simulink model "HMC"  (R2026a)
settings: Solver=ode1  StopTime=inf  FixedStep=0.0001
PreLoadFcn:
  | %load('C:\Users\bme_master\Desktop\mot\mot_6_deneme.mat')
  | 
  | 
  | %load('C:\Users\bme_master\Desktop\mot\PRE_G''s.mat')
PostLoadFcn:
  | , if any(exist('dsrtsu_mdlpostloadfcn', 'file') ~= 0), dsrtsu_mdlpostloadfcn('Execute', bdroot); end,
InitFcn:
  | %motor_control_init_m
  | %clear all
  | %close all
  | %clc
  | b=1e-8
  | StepSize = 1e-4;
  | N=1e-17;
  | 
  | VLV_0 =0;%120; %120
  | VA_0 = 0;%300; %300
  | VRV_0 = 0;%130;
  | VP_0 = 0;%500;
  | VLA_0 = 0;%20;
  | VV_0=5000;
  | VRA_0=0;
  | 
  | 
  | QLV_0 = 0;
  | QLA_0 = 0;
  | QP_0 = 0;
  | 
  | bh = 0;
  | th =0;
  | 
  | X_0 = [VLV_0 VA_0 VV_0 VP_0  VLA_0  VRA_0 VRV_0];
  | 
  | 
  | V0 = 10;
  | 
  | K1=.0004;%0.0001
  | K2=0.0009;%0.0009
  | KA=1;%1
  | C1=0.000000003;%0.0000003
  | lambda=6000;%3000
  | X_00 = [VLV_0 VA_0 VV_0 VRV_0];
  | 
  | r2 = 0.05/2;
  | A2 = pi*r2^2;
  | h2 = 0.63;
  | V2 = A2*h2;
  | 
  | 
  | r3 = 0.05/2;
  | A3 = pi*r3^2;
  | h3 = 0.63;
  | V3 = A3*h3;
  | 
  | 
  | rho = 997;
  | gg = 9.81;
  | %
  | init_min=0;
  | init_max=0;
  | %
  | PWM_Period =  StepSize;
  | PWM_Period_g1 = PWM_Period;
  | PWM_Period_g2 =PWM_Period;
  | PWM_Period_g3 = PWM_Period;
  | PWM_Period_g4 = PWM_Period;
  | PWM_Period_g5 = PWM_Period;
  | ... (+158 lines)
undefined symbols (not defined in the file or in its folder): Continuous, DiscIntNeverNeededParam, Time
libraries: powerlib_meascontrol x19, simulink x15, rti1202lib_adc_class1 x11, cstblocks x10, rti1202lib_dio_class1 x8, dspstat3 x3, rti1202lib_dac_class1 x1, dspswit3 x1, ctrlSharedLib x1, slpidlib x1, dsparch4 x1
(part 3 of 5)

== system HMC/Reference CVSs/Pm/PID ==
  s : Inport
  LTI System : cstblocks/LTI System  sys=tfa  IC=[]
  PID Controller : simulink/Continuous/PID Controller  Controller=PID  Form=Parallel  TimeDomain=Continuous-time  SampleTime=-1  IntegratorMethod=Forward Euler  FilterMethod=Forward Euler  ControllerParametersSource=internal  P=0  I=0.336541519886425  D=0  UseFilter=on  N=100  TunerSelectOption=Transfer Function Based (PID Tuner App)  InitialConditionSource=internal  InitialConditionForIntegrator=0  InitialConditionForFilter=0  DifferentiatorICPrevScaledInput=0  ExternalReset=none  TrackingMode=off  Kt=1  LimitOutput=off  UpperSaturationLimit=inf  LowerSaturationLimit=-inf  LinearizeAsGain=on  AntiWindupMode=none  Kb=1  POutMin=[]  POutMax=[]  IOutMin=[]  IOutMax=[]  DOutMin=[]  DOutMax=[]  NOutMin=[]  NOutMax=[]  SumOutMin=[]  SumOutMax=[]  SaturationOutMin=[]  SaturationOutMax=[]  PParamMin=[]  PParamMax=[]  IParamMin=[]  IParamMax=[]  DParamMin=[]  DParamMax=[]  NParamMin=[]  NParamMax=[]  KbParamMin=[]  KbParamMax=[]  KtParamMin=[]  KtParamMax=[]  KbOutMin=[]  KbOutMax=[]  KtOutMin=[]  KtOutMax=[]  IntegratorOutMin=[]  IntegratorOutMax=[]  FilterOutMin=[]  FilterOutMax=[]  SumI1OutMin=[]  SumI1OutMax=[]  SumI2OutMin=[]  SumI2OutMax=[]  SumI3OutMin=[]  SumI3OutMax=[]  SumI4OutMin=[]  SumI4OutMax=[]  SumDOutMin=[]  SumDOutMax=[]  DifferentiatorOutMin=[]  DifferentiatorOutMax=[]  FilterDiffOutCoefMin=[]  FilterDiffOutCoefMax=[]  ReciprocalOutMin=[]  ReciprocalOutMax=[]  SumDenOutMin=[]  SumDenOutMax=[]  SumNumOutMin=[]  SumNumOutMax=[]  DivideOutMin=[]  DivideOutMax=[]  IntegratorContinuousStateAttributes=''  IntegratorStateMustResolveToSignalObject=off  IntegratorRTWStateStorageClass=Auto  FilterContinuousStateAttributes=''  FilterStateMustResolveToSignalObject=off  FilterRTWStateStorageClass=Auto  ParallelPVariant=InternalParameters  IdealPVariant=Disabled  IVariant=InternalParameters  DVariant=InternalParameters  IntegratorVariant=Continuous  SatVariant=Disabled  AWVariant=Passthrough  PCopyVariant=Disabled  TRVariant=Disabled  FdbkBlocksVariant=Forward  IdealPFdbkVariant=Disabled  SatFdbkVariant=Disabled  DerivativeFilterVariant=ContFilter  NVariant=InternalParameters  NCopyVariant=Disabled  FilterICVariant=InternalICsFilter  IntegratorICVariant=InternalICs  ExternalResetVariant=Disabled  TRSumVariant=Passthrough  SumFdbkVariant=Disabled  SumVariant=Sum_PID
  Sum1 : Sum  Inputs=|+-
  To Workspace : ToWorkspace  VariableName=input  SampleTime=-1
  To Workspace1 : ToWorkspace  VariableName=output  SampleTime=-1
  E : Outport  VectorParamsAs1DForOutWhenUnconnected=off
  wires:
  LTI System/1 -> To Workspace1/1, E/1, Sum1/2
  Sum1/1 -> PID Controller/1
  s/1 -> Sum1/1
  PID Controller/1 -> LTI System/1, To Workspace/1

== system HMC/Reference CVSs/Pressures Flows and Volumes/Exercise ==
  note: y = 0,0167x 2 + 0,6667x + 180
  note: y = -0,0069x2 + 1,2813x + 30,375R² = 1
  note: y = -0,1479x 2 + 38,021x - 923,75
  note: y = 0,1417x 2 - 24,583x + 2165
  note: y = -0,0033x 2 + 0,8667x - 16
  HR1 : Inport
  Enable : EnablePort
  Add{1..10,18..19} (12 alike) : Sum
  Constant1 : Constant  Value=180
  Constant2 : Constant  Value=-923.75
  Constant20 : Constant  Value=0.5621
  Constant3 : Constant  Value=30.375
  Constant4 : Constant  Value=-16
  Constant5 : Constant  Value=2165
  Gain : Gain  Gain=1/10000
  Gain1 : Gain  Gain=0.0167
  Gain10 : Gain  Gain=0.1417
  Gain11 : Gain  Gain=-24.583
  Gain12 : Gain  Gain=1/1000
  Gain13 : Gain  Gain=-0.0069
  Gain14 : Gain  Gain=1.2813
  Gain15 : Gain  Gain=1/10000
  Gain2 : Gain  Gain=0.000003
  Gain3 : Gain  Gain=-0.0008
  Gain4 : Gain  Gain=0.6667
  Gain5 : Gain  Gain=1/10000
  Gain6 : Gain  Gain=-0.0033
  Gain7 : Gain  Gain=0.8667
  Gain8 : Gain  Gain=-0.1479
  Gain9 : Gain  Gain=38.021
  Mux : Mux  Inputs=5
  Product{1..5,15} (6 alike) : Product
  Output : Outport
  wires:
  Add19/1 -> Mux/5  "eA"
  Product15/1 -> Gain2/1
  Constant20/1 -> Add19/2
  Add18/1 -> Add19/1
  Gain3/1 -> Add18/2
  Gain2/1 -> Add18/1
  Constant1/1 -> Add2/2
  HR1/1 -> Product2/1, Gain9/1, Product2/2, Product4/1, Product4/2, Gain14/1, Product5/1, Product5/2, Product15/1, Product15/2, Gain3/1, Gain4/1, Product1/2, Product1/1, Gain11/1, Gain7/1, Product3/2, Product3/1
  Add1/1 -> Add2/1
  Product1/1 -> Gain1/1
  Gain1/1 -> Add1/1
  Gain4/1 -> Add1/2
  Mux/1 -> Output/1
  Gain10/1 -> Add9/1
  Constant5/1 -> Add10/2
  Gain11/1 -> Add9/2
  Add9/1 -> Add10/1
  Add3/1 -> Add6/1
  Gain9/1 -> Add3/2
  Gain8/1 -> Add3/1
  Product4/1 -> Gain13/1
  Add8/1 -> Gain12/1
  Gain12/1 -> Mux/3
  Add10/1 -> Gain15/1
  Constant3/1 -> Add8/2
  Gain13/1 -> Add7/1
  Constant4/1 -> Add5/2
  Add4/1 -> Add5/1
  Gain6/1 -> Add4/1
  Constant2/1 -> Add6/2
  Add6/1 -> Gain/1
  Add5/1 -> Gain5/1
  Product2/1 -> Gain8/1
  Add7/1 -> Add8/1
  Gain5/1 -> Mux/1
  Product3/1 -> Gain6/1
  Gain14/1 -> Add7/2
  Gain7/1 -> Add4/2
  Product5/1 -> Gain10/1
  Gain/1 -> Mux/2
  Gain15/1 -> Mux/4

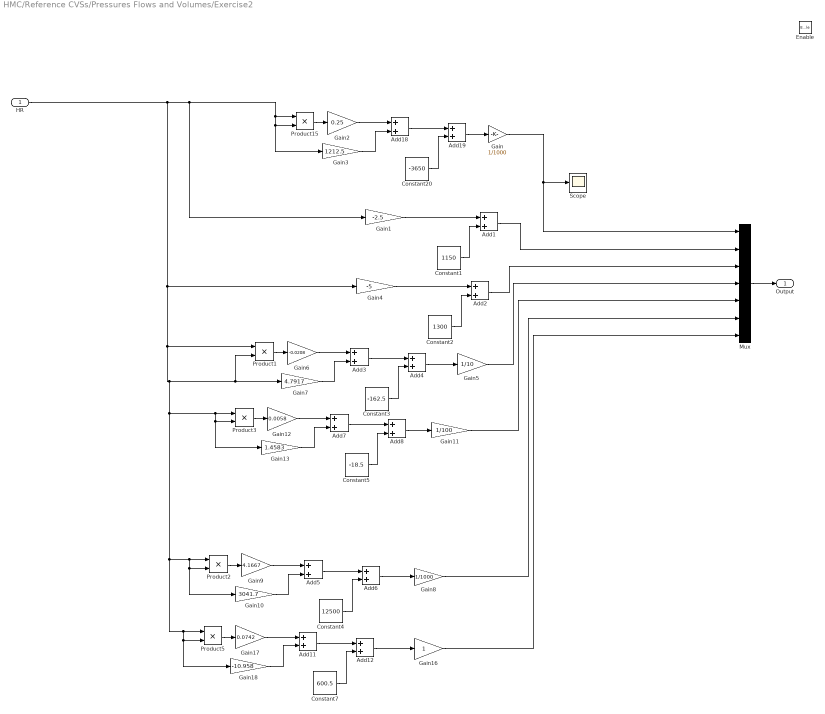
== system HMC/Reference CVSs/Pressures Flows and Volumes/Exercise2 ==
  HR : Inport
  Enable : EnablePort
  Add{1..8,11..12,18..19} (12 alike) : Sum
  Constant1 : Constant  Value=1150
  Constant2 : Constant  Value=1300
  Constant20 : Constant  Value=-3650
  Constant3 : Constant  Value=-162.5
  Constant4 : Constant  Value=12500
  Constant5 : Constant  Value=-18.5
  Constant7 : Constant  Value=600.5
  Gain : Gain  Gain=1/1000
  Gain1 : Gain  Gain=-2.5
  Gain10 : Gain  Gain=3041.7
  Gain11 : Gain  Gain=1/100
  Gain12 : Gain  Gain=0.0058
  Gain13 : Gain  Gain=1.4583
  Gain16 : Gain
  Gain17 : Gain  Gain=0.0742
  Gain18 : Gain  Gain=-10.958
  Gain2 : Gain  Gain=0.25
  Gain3 : Gain  Gain=1212.5
  Gain4 : Gain  Gain=-5
  Gain5 : Gain  Gain=1/10
  Gain6 : Gain  Gain=-0.0208
  Gain7 : Gain  Gain=4.7917
  Gain8 : Gain  Gain=1/1000
  Gain9 : Gain  Gain=4.1667
  Mux : Mux  Inputs=7
  Product{1..3,5,15} (5 alike) : Product
  Scope : Scope
      settings: ActiveDisplayYMinimum=60  ActiveDisplayYMaximum=80  DataLoggingVariableName=ScopeData9
  Output : Outport
  wires:
  Gain9/1 -> Add5/1
  Product2/1 -> Gain9/1
  Add5/1 -> Add6/1
  Gain8/1 -> Mux/6
  Gain10/1 -> Add5/2
  Constant4/1 -> Add6/2
  Add6/1 -> Gain8/1
  Add3/1 -> Add4/1
  Add4/1 -> Gain5/1
  Gain6/1 -> Add3/1
  Product1/1 -> Gain6/1
  Gain5/1 -> Mux/4
  Gain7/1 -> Add3/2
  Constant3/1 -> Add4/2
  Constant2/1 -> Add2/2
  Add2/1 -> Mux/3
  Gain4/1 -> Add2/1
  Gain1/1 -> Add1/1
  Constant1/1 -> Add1/2
  Add1/1 -> Mux/2
  Add18/1 -> Add19/1
  Add19/1 -> Gain/1
  Gain3/1 -> Add18/2
  Product15/1 -> Gain2/1
  Constant20/1 -> Add19/2
  Gain/1 -> Scope/1, Mux/1
  Gain2/1 -> Add18/1
  Mux/1 -> Output/1
  Gain12/1 -> Add7/1
  Add7/1 -> Add8/1
  Constant5/1 -> Add8/2
  Product3/1 -> Gain12/1
  Add8/1 -> Gain11/1
  Gain11/1 -> Mux/5
  Gain13/1 -> Add7/2
  Product5/1 -> Gain17/1
  Add11/1 -> Add12/1
  Constant7/1 -> Add12/2
  Add12/1 -> Gain16/1
  HR/1 -> Gain3/1, Product15/2, Product15/1, Gain1/1, Gain7/1, Product1/2, Gain10/1, Product2/2, Product2/1, Product5/1, Product5/2, Gain18/1, Gain13/1, Product3/2, Product3/1, Product1/1, Gain4/1
  Gain17/1 -> Add11/1
  Gain16/1 -> Mux/7
  Gain18/1 -> Add11/2

== system HMC/Reference CVSs/Pressures Flows and Volumes/HF ==
  note: y = 0,5x + 40
  note: y = - 0,3333x + 130
  note: y = 0,0128x 2 - 1,9167x + 179
  note: y = -0,0189x 2 + 3,5x + 78
  note: y = 0,4333x + 14
  note: eV
  note: eRA
  note: eLA
  note: eP
  note: eA
  HR : Inport
  Enable : EnablePort
  Add{1..4,6,8,19} (7 alike) : Sum
  Constant1 : Constant  Value=78
  Constant2 : Constant  Value=179
  Constant20 : Constant  Value=14
  Constant3 : Constant  Value=130
  Constant4 : Constant  Value=40
  Gain : Gain  Gain=1/1000
  Gain1 : Gain  Gain=1/10000
  Gain11 : Gain  Gain=-0.3333
  Gain13 : Gain  Gain=0.5
  Gain3 : Gain  Gain=0.4333
  Gain4 : Gain  Gain=-0.0189
  Gain5 : Gain  Gain=3.5
  Gain6 : Gain  Gain=1/1000
  Gain7 : Gain  Gain=0.0128
  Gain8 : Gain  Gain=-1.9167
  Gain9 : Gain  Gain=1/1000
  Multiply : Gain  Gain=1/100
  Mux : Mux  Inputs=5
  Product1 : Product
  Product2 : Product
  Output : Outport
  wires:
  Gain3/1 -> Add19/1
  Constant20/1 -> Add19/2
  Gain1/1 -> Mux/1
  Add19/1 -> Gain1/1
  Add1/1 -> Add2/1
  Gain/1 -> Mux/2
  Product1/1 -> Gain4/1
  Gain4/1 -> Add1/1
  Add2/1 -> Gain/1
  Gain5/1 -> Add1/2
  Constant1/1 -> Add2/2
  Add3/1 -> Add4/1
  Gain7/1 -> Add3/1
  Gain8/1 -> Add3/2
  Add4/1 -> Gain6/1
  Constant2/1 -> Add4/2
  Product2/1 -> Gain7/1
  Gain6/1 -> Mux/3
  Add6/1 -> Gain9/1
  Gain11/1 -> Add6/1
  Constant3/1 -> Add6/2
  Gain9/1 -> Mux/4
  Mux/1 -> Output/1
  Multiply/1 -> Mux/5
  Add8/1 -> Multiply/1
  Constant4/1 -> Add8/2
  Gain13/1 -> Add8/1
  HR/1 -> Product1/1, Product1/2, Gain5/1, Gain13/1, Gain11/1, Product2/1, Product2/2, Gain8/1, Gain3/1

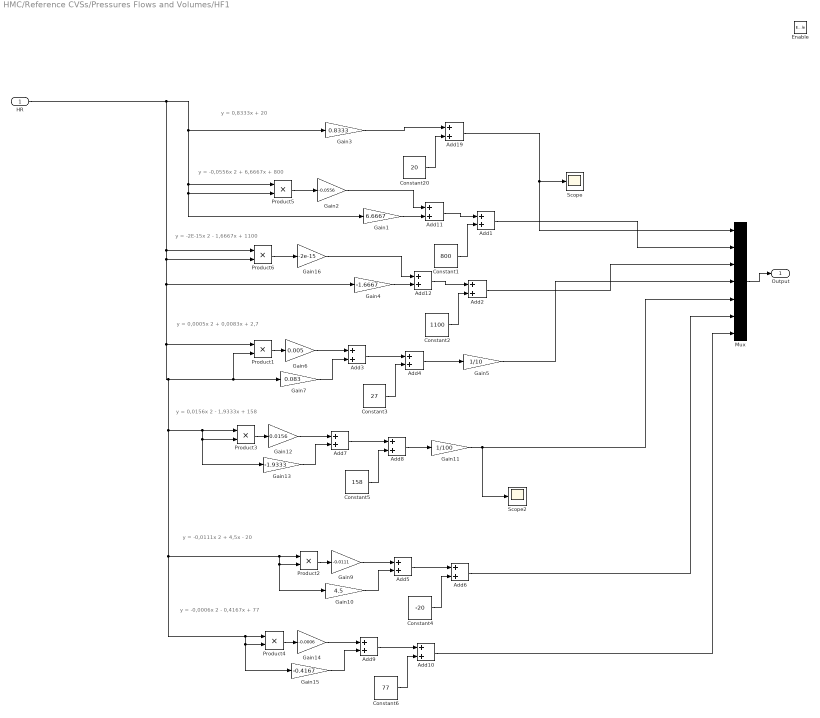
== system HMC/Reference CVSs/Pressures Flows and Volumes/HF1 ==
  note: y = -0,0111x 2 + 4,5x - 20
  note: y = -2E-15x 2 - 1,6667x + 1100
  note: y = 0,8333x + 20
  note: y = 0,0005x 2 + 0,0083x + 2,7
  note: y = -0,0556x 2 + 6,6667x + 800
  note: y = 0,0156x 2 - 1,9333x + 158
  note: y = -0,0006x 2 - 0,4167x + 77
  HR : Inport
  Enable : EnablePort
  Add{1..12,19} (13 alike) : Sum
  Constant1 : Constant  Value=800
  Constant2 : Constant  Value=1100
  Constant20 : Constant  Value=20
  Constant3 : Constant  Value=27
  Constant4 : Constant  Value=-20
  Constant5 : Constant  Value=158
  Constant6 : Constant  Value=77
  Gain1 : Gain  Gain=6.6667
  Gain10 : Gain  Gain=4.5
  Gain11 : Gain  Gain=1/100
  Gain12 : Gain  Gain=0.0156
  Gain13 : Gain  Gain=-1.9333
  Gain14 : Gain  Gain=-0.0006
  Gain15 : Gain  Gain=-0.4167
  Gain16 : Gain  Gain=-2e-15
  Gain2 : Gain  Gain=-0.0556
  Gain3 : Gain  Gain=0.8333
  Gain4 : Gain  Gain=-1.6667
  Gain5 : Gain  Gain=1/10
  Gain6 : Gain  Gain=0.005
  Gain7 : Gain  Gain=0.083
  Gain9 : Gain  Gain=-0.0111
  Mux : Mux  Inputs=7
  Product{1..6} (6 alike) : Product
  Scope : Scope
      settings: ActiveDisplayYMinimum=60  ActiveDisplayYMaximum=80  DataLoggingVariableName=ScopeData4
  Scope2 : Scope
      settings: ActiveDisplayYMinimum=0.88246  ActiveDisplayYMaximum=1.08246  DataLoggingVariableName=ScopeData5
  Output : Outport
  wires:
  Add6/1 -> Mux/6
  Product6/1 -> Gain16/1
  Product5/1 -> Gain2/1
  Gain1/1 -> Add11/2
  Add4/1 -> Gain5/1
  Product4/1 -> Gain14/1
  Gain13/1 -> Add7/2
  Constant6/1 -> Add10/2
  Gain12/1 -> Add7/1
  Gain16/1 -> Add12/1
  Add2/1 -> Mux/3
  Constant3/1 -> Add4/2
  Gain10/1 -> Add5/2
  Gain9/1 -> Add5/1
  Gain11/1 -> Mux/5, Scope2/1
  Product1/1 -> Gain6/1
  Add8/1 -> Gain11/1
  Gain7/1 -> Add3/2
  Add7/1 -> Add8/1
  Product2/1 -> Gain9/1
  Constant4/1 -> Add6/2
  Gain6/1 -> Add3/1
  Constant2/1 -> Add2/2
  Mux/1 -> Output/1
  Constant1/1 -> Add1/2
  Product3/1 -> Gain12/1
  Gain14/1 -> Add9/1
  Add9/1 -> Add10/1
  Gain15/1 -> Add9/2
  Gain3/1 -> Add19/1
  Add19/1 -> Mux/1, Scope/1
  Constant5/1 -> Add8/2
  Gain5/1 -> Mux/4
  Add10/1 -> Mux/7
  Add11/1 -> Add1/1
  Add3/1 -> Add4/1
  Add1/1 -> Mux/2
  Gain4/1 -> Add12/2
  Constant20/1 -> Add19/2
  Gain2/1 -> Add11/1
  Add5/1 -> Add6/1
  Add12/1 -> Add2/1
  HR/1 -> Product6/1, Product6/2, Gain4/1, Product1/1, Gain13/1, Product3/2, Product3/1, Gain15/1, Product4/2, Product4/1, Product2/1, Product2/2, Gain10/1, Product1/2, Gain7/1, Product5/1, Gain1/1, Product5/2, Gain3/1

== system HMC/Reference CVSs/Pressures Flows and Volumes/Rest ==
  note: eC
  note: y = -0,0033x 2 + 0,8667x - 16
  note: eRA
  note: eLA
  note: eP
  note: y = 0,1417x 2 - 24,583x + 2165
  note: y = -0,0069x2 + 1,2813x + 30,375R² = 1
  note: y = -0,1479x 2 + 38,021x - 923,75
  note: y = 0,5x + 40
  note: eV
  HR : Inport
  Input : Inport  Port=2
  Enable : EnablePort
  Add{1..7,18..19} (9 alike) : Sum
  Constant1 : Constant  Value=-923.75
  Constant2 : Constant  Value=30.375
  Constant20 : Constant  Value=-16
  Constant3 : Constant  Value=2165
  Constant4 : Constant  Value=40
  Gain : Gain  Gain=1/10000
  Gain1 : Gain  Gain=1/10000
  Gain10 : Gain  Gain=0.1417
  Gain11 : Gain  Gain=-24.583
  Gain12 : Gain  Gain=1/100
  Gain13 : Gain  Gain=0.5
  Gain2 : Gain  Gain=-0.0033
  Gain3 : Gain  Gain=0.8667
  Gain4 : Gain  Gain=-0.1479
  Gain5 : Gain  Gain=38.021
  Gain6 : Gain  Gain=1/1000
  Gain7 : Gain  Gain=-0.0069
  Gain8 : Gain  Gain=1.2813
  Gain9 : Gain  Gain=1/10000
  Mux : Mux  Inputs=5
  Product{1..3,15} (4 alike) : Product
  Output : Outport
  wires:
  Gain3/1 -> Add18/2
  Product15/1 -> Gain2/1
  Add19/1 -> Gain1/1
  Constant20/1 -> Add19/2
  Gain2/1 -> Add18/1
  Add18/1 -> Add19/1
  Gain1/1 -> Mux/1
  Gain6/1 -> Mux/3
  Mux/1 -> Output/1
  Gain/1 -> Mux/2
  Gain9/1 -> Mux/4
  Gain4/1 -> Add1/1
  Gain5/1 -> Add1/2
  Constant1/1 -> Add2/2
  Add2/1 -> Gain/1
  Add1/1 -> Add2/1
  Product1/1 -> Gain4/1
  Gain7/1 -> Add3/1
  Constant2/1 -> Add4/2
  Add3/1 -> Add4/1
  Add4/1 -> Gain6/1
  Gain8/1 -> Add3/2
  Product2/1 -> Gain7/1
  HR/1 -> Product1/1, Gain5/1, Product1/2, Product2/1, Product2/2, Gain8/1, Product3/1, Product3/2, Gain11/1, Gain3/1, Product15/2, Product15/1
  Add5/1 -> Add6/1
  Product3/1 -> Gain10/1
  Constant3/1 -> Add6/2
  Gain10/1 -> Add5/1
  Gain11/1 -> Add5/2
  Add6/1 -> Gain9/1
  Add7/1 -> Gain12/1
  Constant4/1 -> Add7/2
  Gain13/1 -> Add7/1
  Gain12/1 -> Mux/5  "eA"
  Input/1 -> Gain13/1

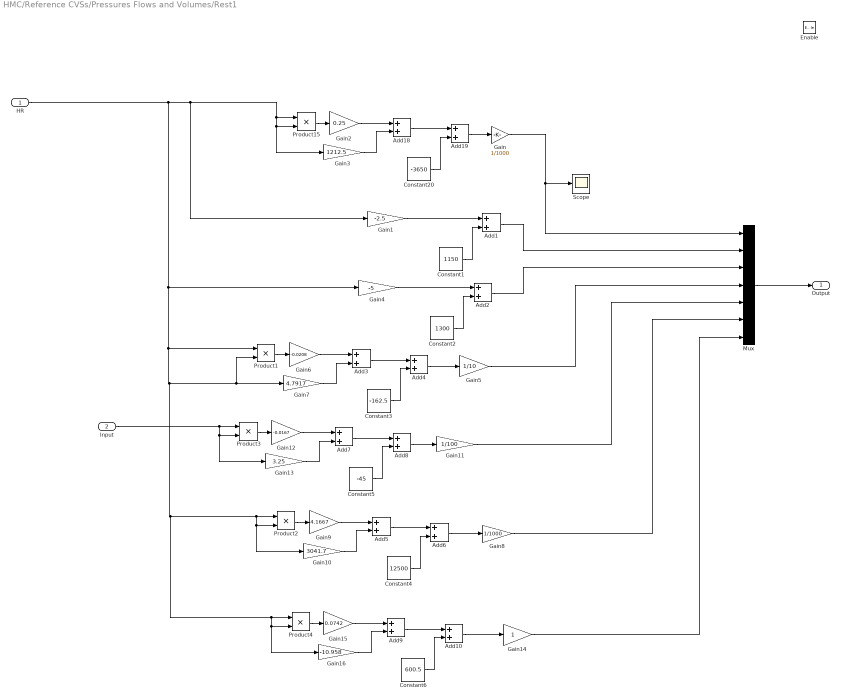
== system HMC/Reference CVSs/Pressures Flows and Volumes/Rest1 ==
  HR : Inport
  Input : Inport  Port=2
  Enable : EnablePort
  Add{1..10,18..19} (12 alike) : Sum
  Constant1 : Constant  Value=1150
  Constant2 : Constant  Value=1300
  Constant20 : Constant  Value=-3650
  Constant3 : Constant  Value=-162.5
  Constant4 : Constant  Value=12500
  Constant5 : Constant  Value=-45
  Constant6 : Constant  Value=600.5
  Gain : Gain  Gain=1/1000
  Gain1 : Gain  Gain=-2.5
  Gain10 : Gain  Gain=3041.7
  Gain11 : Gain  Gain=1/100
  Gain12 : Gain  Gain=-0.0167
  Gain13 : Gain  Gain=3.25
  Gain14 : Gain
  Gain15 : Gain  Gain=0.0742
  Gain16 : Gain  Gain=-10.958
  Gain2 : Gain  Gain=0.25
  Gain3 : Gain  Gain=1212.5
  Gain4 : Gain  Gain=-5
  Gain5 : Gain  Gain=1/10
  Gain6 : Gain  Gain=-0.0208
  Gain7 : Gain  Gain=4.7917
  Gain8 : Gain  Gain=1/1000
  Gain9 : Gain  Gain=4.1667
  Mux : Mux  Inputs=7
  Product{1..4,15} (5 alike) : Product
  Scope : Scope
      settings: ActiveDisplayYMinimum=60  ActiveDisplayYMaximum=80  DataLoggingVariableName=ScopeData9
  Output : Outport
  wires:
  Mux/1 -> Output/1
  Gain2/1 -> Add18/1
  Gain/1 -> Mux/1, Scope/1
  Constant20/1 -> Add19/2
  Product15/1 -> Gain2/1
  Gain3/1 -> Add18/2
  Add19/1 -> Gain/1
  Add18/1 -> Add19/1
  Add1/1 -> Mux/2
  Constant1/1 -> Add1/2
  Gain1/1 -> Add1/1
  Gain4/1 -> Add2/1
  Add2/1 -> Mux/3
  Constant2/1 -> Add2/2
  Constant3/1 -> Add4/2
  Gain7/1 -> Add3/2
  Gain5/1 -> Mux/4
  Product1/1 -> Gain6/1
  Gain6/1 -> Add3/1
  Add4/1 -> Gain5/1
  Add3/1 -> Add4/1
  Add6/1 -> Gain8/1
  Constant4/1 -> Add6/2
  Gain10/1 -> Add5/2
  Gain8/1 -> Mux/6
  Add5/1 -> Add6/1
  Product2/1 -> Gain9/1
  Gain9/1 -> Add5/1
  Gain13/1 -> Add7/2
  Add7/1 -> Add8/1
  Product3/1 -> Gain12/1
  Constant5/1 -> Add8/2
  Add8/1 -> Gain11/1
  Gain12/1 -> Add7/1
  Input/1 -> Product3/1, Product3/2, Gain13/1
  Gain11/1 -> Mux/5
  Product4/1 -> Gain15/1
  Add9/1 -> Add10/1
  Constant6/1 -> Add10/2
  Add10/1 -> Gain14/1
  HR/1 -> Gain4/1, Product1/1, Product4/1, Product4/2, Gain16/1, Product2/1, Product2/2, Gain10/1, Product1/2, Gain7/1, Gain1/1, Product15/1, Product15/2, Gain3/1
  Gain15/1 -> Add9/1
  Gain14/1 -> Mux/7
  Gain16/1 -> Add9/2

== system HMC/Reference CVSs/Pressures Flows and Volumes/Subsystem13 ==
  note: y = 0,0083x 2 - 0,9167x + 40
  note: y = 0,1944x 2 - 28,333x + 1100
  Add{1..2,18..19} (4 alike) : Sum
  Constant1 : Constant  Value=40
  Constant20 : Constant  Value=1100
  Display : Display
  Gain : Gain  Gain=1/10
  Gain2 : Gain  Gain=0.1944
  Gain3 : Gain  Gain=-28.333
  Gain4 : Gain  Gain=0.0083
  Gain5 : Gain  Gain=-0.9167
  Product1 : Product
  Product15 : Product
  Scope : Scope
      settings: ActiveDisplayYMinimum=8.99968  ActiveDisplayYMaximum=10.99968  DataLoggingVariableName=ScopeData2
  Scope1 : Scope
      settings: ActiveDisplayYMinimum=8.99968  ActiveDisplayYMaximum=10.99968
  Switch : Switch  Criteria=u2 > Threshold  SaturateOnIntegerOverflow=off  InputSameDT=off
  V0 : Outport
  wires:
  Add19/1 -> Gain/1
  Add18/1 -> Add19/1
  Gain3/1 -> Add18/2
  Product15/1 -> Gain2/1
  Constant20/1 -> Add19/2
  Gain2/1 -> Add18/1
  [HR] -> Product15/1, Product15/2, Gain3/1
  Gain/1 -> Switch/3, Scope/1
  Add2/1 -> Switch/1, Scope1/1
  [HR] -> Gain5/1, Product1/2, Product1/1
  Gain4/1 -> Add1/1
  Constant1/1 -> Add2/2
  Product1/1 -> Gain4/1
  Gain5/1 -> Add1/2
  Add1/1 -> Add2/1
  [Heart_Failure_On_Off] -> Switch/2
  Switch/1 -> Display/1, V0/1

== system HMC/Reference CVSs/Pressures Flows and Volumes/Subsystem5 ==
  In1 : Inport
  elv : Inport  Port=2
  erv : Inport  Port=3
  In4 : Inport  Port=4
  Switch : Switch  Criteria=u2 > Threshold  SaturateOnIntegerOverflow=off  InputSameDT=off
  Switch4 : Switch  Criteria=u2 > Threshold  SaturateOnIntegerOverflow=off  InputSameDT=off
  VolumesForVAD : Subsystem
  Out1 : Outport
  Output1 : Outport  Port=2
  wires:
  [QVAD] -> Switch4/2, Switch/2
  elv/1 -> VolumesForVAD/1(elv1)
  VolumesForVAD/2(Output1) -> Switch4/1
  erv/1 -> VolumesForVAD/2(erv1)
  VolumesForVAD/1(Output2) -> Switch/1
  In1/1 -> Switch/3
  Switch4/1 -> Output1/1
  Switch/1 -> Out1/1
  In4/1 -> Switch4/3

== system HMC/Reference CVSs/eLV/LV_e_min ==
  VLV : Inport
  Add : Sum  Inputs=+-
  Add1 : Sum  Inputs=+-
  Add2 : Sum
  Constant9 : Constant
  Display : Display
  Display1 : Display
  Exp : Math  SignedPower=on
  Product : Product
  Product1 : Product
  Real_CLV : Subsystem
  Subsystem1 : Subsystem
  Subsystem2 : Subsystem
  Subsystem5 : Subsystem
  Switch : Switch  Criteria=u2 > Threshold  SaturateOnIntegerOverflow=off  InputSameDT=off
  Switch1 : Switch  Criteria=u2 > Threshold  SaturateOnIntegerOverflow=off  InputSameDT=off
  Switch2 : Switch  Criteria=u2 > Threshold  SaturateOnIntegerOverflow=off  InputSameDT=off
  a_LV_Cons : Constant  Value=0.4641
  d_LV_Cons : Constant  Value=0.1235
  resting : Subsystem
  eLV_min_O : Outport
  tag scope: bLV=global, cLV=global
  wires:
  Add/1 -> Product1/2
  Product1/1 -> Exp/1
  Exp/1 -> Add1/1
  d_LV_Cons/1 -> Add2/2
  Product/1 -> Add2/1
  Add1/1 -> Product/2
  Constant9/1 -> Add1/2
  VLV/1 -> Add/1
  Add2/1 -> eLV_min_O/1
  a_LV_Cons/1 -> Product/1
  [Heart_Failure_On_Off] -> Switch/2
  Subsystem1/1(C_LV) -> Switch1/3
  [Heart_Failure_On_Off] -> Switch1/2
  Real_CLV/1(C_LV) -> Switch1/1
  Subsystem5/1(B_LV_HF) -> Switch/1
  [Exercise_On_Off] -> Switch2/2
  resting/1(B_LV) -> Switch2/3
  Subsystem2/1(B_LV) -> Switch2/1
  Switch/1 -> [bLV], Product1/1, Display/1
  Switch2/1 -> Switch/3
  Switch1/1 -> [cLV], Add/2, Display1/1

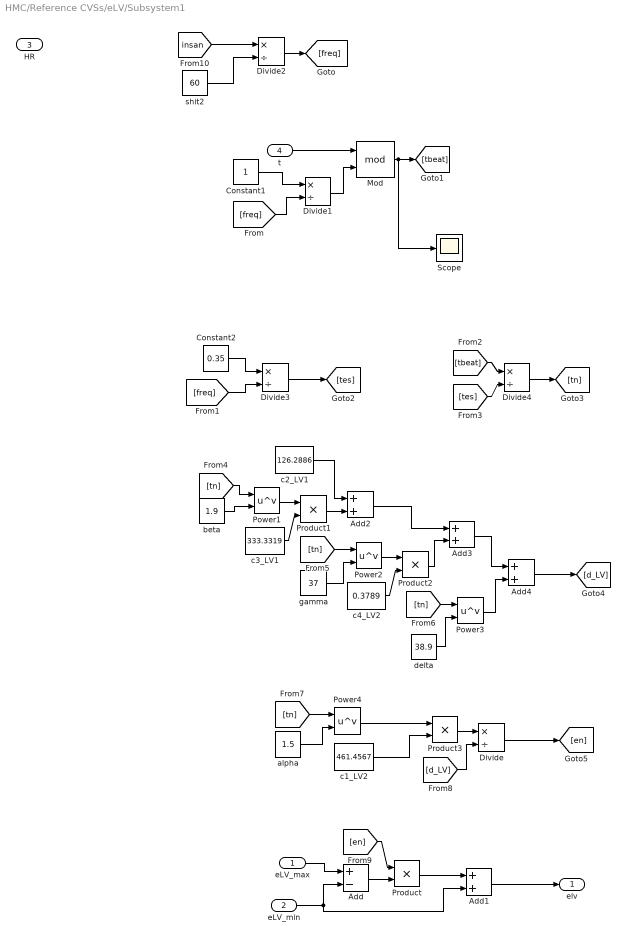
== system HMC/Reference CVSs/eLV/Subsystem1 ==
  eLV_max : Inport
  eLV_min : Inport  Port=2
  HR : Inport  Port=3
  t : Inport  Port=4
  Add : Sum  Inputs=+-
  Add{1..4} (4 alike) : Sum
  Constant1 : Constant
  Constant2 : Constant  Value=0.35
  Divide{,1..4} (5 alike) : Product  Inputs=*/  RndMeth=Zero  SaturateOnIntegerOverflow=on
  Mod : Math  Operator=mod  SignedPower=on
  Power{1..4} (4 alike) : Math  Operator=pow  SignedPower=on
  Product{,1..3} (4 alike) : Product
  Scope : Scope
      settings: ActiveDisplayYMinimum=-0.05357  ActiveDisplayYMaximum=0.43719  DataLoggingVariableName=ScopeData4
  alpha : Constant  Value=1.5
  beta : Constant  Value=1.9
  c1_LV2 : Constant  Value=461.4567
  c2_LV1 : Constant  Value=126.2886
  c3_LV1 : Constant  Value=333.3319
  c4_LV2 : Constant  Value=0.3789
  delta : Constant  Value=38.9
  gamma : Constant  Value=37
  "shit2 " : Constant  Value=60
  elv : Outport
  wires:
  Product/1 -> Add1/1
  Add/1 -> Product/2
  Add1/1 -> elv/1
  eLV_min/1 -> Add/2, Add1/2
  eLV_max/1 -> Add/1
  "shit2 "/1 -> Divide2/2
  Divide2/1 -> [freq]
  [freq] -> Divide1/2
  Constant1/1 -> Divide1/1
  Constant2/1 -> Divide3/1
  [freq] -> Divide3/2
  Divide3/1 -> [tes]
  [tbeat] -> Divide4/1
  [tes] -> Divide4/2
  Divide4/1 -> [tn]
  c2_LV1/1 -> Add2/1
  [tn] -> Power1/1
  beta/1 -> Power1/2
  Power1/1 -> Product1/1
  c3_LV1/1 -> Product1/2
  Product1/1 -> Add2/2
  Add2/1 -> Add3/1
  [tn] -> Power2/1
  gamma/1 -> Power2/2
  Power2/1 -> Product2/1
  c4_LV2/1 -> Product2/2
  Product2/1 -> Add3/2
  [tn] -> Power3/1
  delta/1 -> Power3/2
  Add3/1 -> Add4/1
  Power3/1 -> Add4/2
  Add4/1 -> [d_LV]
  [tn] -> Power4/1
  alpha/1 -> Power4/2
  Power4/1 -> Product3/1
  c1_LV2/1 -> Product3/2
  Product3/1 -> Divide/1
  Divide/1 -> [en]
  [d_LV] -> Divide/2
  [en] -> Product/1
  t/1 -> Mod/1
  Divide1/1 -> Mod/2
  Mod/1 -> Scope/1, [tbeat]
  [insan] -> Divide2/1

== system HMC/Reference CVSs/eLV/eLV1 ==
  note: y = 0,0027x 2 - 0,0767x + 24,76
  Add18 : Sum
  Add19 : Sum
  Constant20 : Constant  Value=24.76
  Gain1 : Gain  Gain=1/10
  Gain2 : Gain  Gain=0.0027
  Gain3 : Gain  Gain=-0.0767
  PID : Subsystem  Commented=on
  Product15 : Product
  Scope : Scope
      settings: ActiveDisplayYMinimum=2.20237  ActiveDisplayYMaximum=2.60692
  Stair Generator : powerlib_meascontrol/Pulse & Signal Generators/Stair Generator  Commented=on  t=[0,50,100,150]  e=[3.25,3.5,3.75,4]  Ts=stepsize
      settings: SourceProductName=Simscape Electrical
  Stair Generator1 : powerlib_meascontrol/Pulse & Signal Generators/Stair Generator  Commented=on  t=[100,200,300,400]  e=[3.25,3.5,3.75,4]  Ts=stepsize
      settings: SourceProductName=Simscape Electrical
  Output : Outport
  wires:
  Stair Generator1/1 -> PID/1(s)
  Add19/1 -> Gain1/1
  Gain2/1 -> Add18/1
  Gain3/1 -> Add18/2
  [HR] -> Product15/1, Product15/2, Gain3/1
  Add18/1 -> Add19/1
  Product15/1 -> Gain2/1
  Constant20/1 -> Add19/2
  Gain1/1 -> Scope/1, Output/1

== system HMC/Reference CVSs/eLV/eLVsick ==
  note: y = -0,0028x 2 + 0,9167x + 45
  Add18 : Sum
  Add19 : Sum
  Constant20 : Constant  Value=45
  Gain1 : Gain  Gain=1/100
  Gain2 : Gain  Gain=-0.0028
  Gain3 : Gain  Gain=0.9167
  Product15 : Product
  Scope : Scope
      settings: ActiveDisplayYMinimum=2.20237  ActiveDisplayYMaximum=2.60692  DataLoggingVariableName=ScopeData6
  Output : Outport
  wires:
  Product15/1 -> Gain2/1
  Gain1/1 -> Scope/1, Output/1
  Gain3/1 -> Add18/2
  Constant20/1 -> Add19/2
  Gain2/1 -> Add18/1
  [HR] -> Product15/1, Product15/2, Gain3/1
  Add18/1 -> Add19/1
  Add19/1 -> Gain1/1

== system HMC/Reference CVSs/eRV/RV_e_min ==
  VRV : Inport
  Add3 : Sum  Inputs=+-
  Add4 : Sum
  Constant13 : Constant
  Display1 : Display
  Exp1 : Math  SignedPower=on
  Product2 : Product
  Product3 : Product
  Switch1 : Switch  Criteria=u2 > Threshold  Threshold=0.9  SaturateOnIntegerOverflow=off  InputSameDT=off
  a_RV_Cons : Constant  Value=0.03752
  b_RV_Cons : Constant  Value=0.03776
  c_RV : Subsystem
  real_c_RV : Subsystem
  eRV_min_O : Outport
  tag scope: cRV=global
  wires:
  Constant13/1 -> Add4/2
  Product2/1 -> Exp1/1
  Add3/1 -> Product2/1
  VRV/1 -> Add3/1
  Exp1/1 -> Add4/1
  Add4/1 -> Product3/2
  Switch1/1 -> Display1/1, Add3/2, [cRV]
  a_RV_Cons/1 -> Product3/1
  b_RV_Cons/1 -> Product2/2
  Product3/1 -> eRV_min_O/1
  real_c_RV/1(Output) -> Switch1/1
  [Heart_Failure_On_Off] -> Switch1/2
  c_RV/1(Output) -> Switch1/3

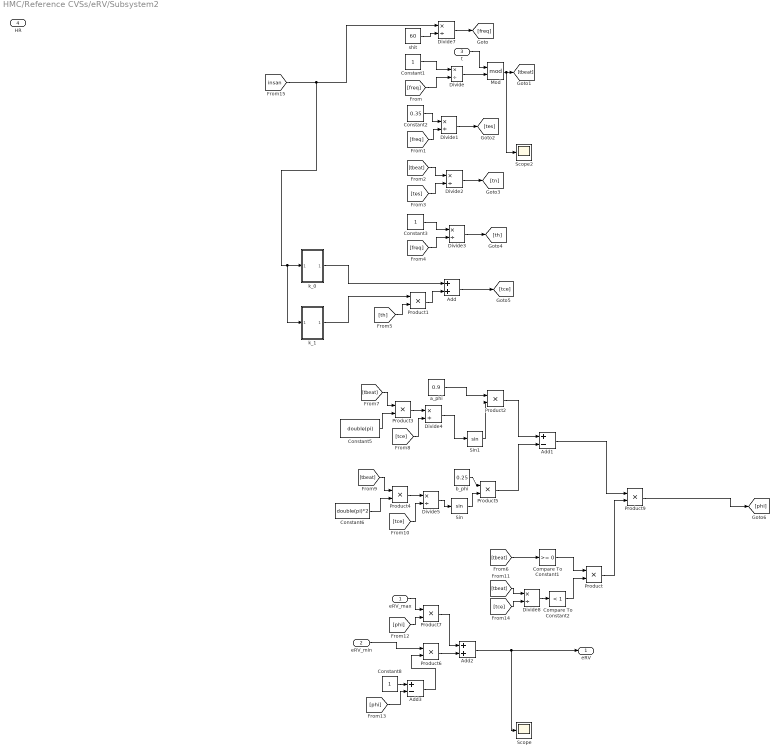
== system HMC/Reference CVSs/eRV/Subsystem2 ==
  eRV_max : Inport
  eRV_min : Inport  Port=2
  t : Inport  Port=3
  HR : Inport  Port=4
  Add : Sum
  Add1 : Sum  Inputs=+-
  Add2 : Sum
  Add3 : Sum  Inputs=+-
  Compare To Constant1 : simulink/Logic and Bit Operations/Compare To Constant  relop=>=  const=0  OutDataTypeStr=boolean
  Compare To Constant2 : simulink/Logic and Bit Operations/Compare To Constant  relop=<  const=1  OutDataTypeStr=boolean
  Constant1 : Constant
  Constant2 : Constant  Value=0.35
  Constant3 : Constant
  Constant5 : Constant  Value=double(pi)
  Constant6 : Constant  Value=double(pi)*2
  Constant8 : Constant
  Divide{,1..5,7..8} (8 alike) : Product  Inputs=*/  RndMeth=Zero  SaturateOnIntegerOverflow=on
  Mod : Math  Operator=mod  SignedPower=on
  Product{,1..7,9} (9 alike) : Product
  Scope : Scope
      settings: ActiveDisplayYMinimum=-0.03117  ActiveDisplayYMaximum=2.17237  DataLoggingVariableName=ScopeData3
  Scope2 : Scope
      settings: ActiveDisplayYMinimum=-0.09374  ActiveDisplayYMaximum=0.84364  DataLoggingVariableName=ScopeData6
  Sin : Trigonometry
  Sin1 : Trigonometry
  a_phi : Constant  Value=0.9
  b_phi : Constant  Value=0.25
  k_0 : Subsystem
  k_1 : Subsystem
  shit : Constant  Value=60
  eRV : Outport
  wires:
  shit/1 -> Divide7/2
  Divide7/1 -> [freq]
  Constant1/1 -> Divide/1
  [freq] -> Divide/2
  Mod/1 -> Scope2/1, [tbeat]
  Constant2/1 -> Divide1/1
  [freq] -> Divide1/2
  Divide1/1 -> [tes]
  [tbeat] -> Divide2/1
  [tes] -> Divide2/2
  Divide2/1 -> [tn]
  Constant3/1 -> Divide3/1
  [freq] -> Divide3/2
  Divide3/1 -> [th]
  [th] -> Product1/2
  Add/1 -> [tce]
  Product1/1 -> Add/2
  [tbeat] -> Compare To Constant1/1
  a_phi/1 -> Product2/1
  [tbeat] -> Product3/1
  Constant5/1 -> Product3/2
  Product3/1 -> Divide4/1
  [tce] -> Divide4/2
  Product2/1 -> Add1/1
  Divide5/1 -> Sin/1
  Constant6/1 -> Product4/2
  [tce] -> Divide5/2
  [tbeat] -> Product4/1
  Product4/1 -> Divide5/1
  Sin/1 -> Product5/2
  b_phi/1 -> Product5/1
  Product5/1 -> Add1/2
  Add1/1 -> Product9/1
  Product9/1 -> [phi]
  eRV_min/1 -> Product6/1
  Product6/1 -> Add2/2
  eRV_max/1 -> Product7/1
  [phi] -> Product7/2
  Product7/1 -> Add2/1
  Add2/1 -> Scope/1, eRV/1
  Constant8/1 -> Add3/1
  [phi] -> Add3/2
  Add3/1 -> Product6/2
  Divide/1 -> Mod/2
  t/1 -> Mod/1
  [tbeat] -> Divide8/1
  [tce] -> Divide8/2
  Divide8/1 -> Compare To Constant2/1
  Compare To Constant1/1 -> Product/1
  Compare To Constant2/1 -> Product/2
  Product/1 -> Product9/2
  Divide4/1 -> Sin1/1
  Sin1/1 -> Product2/2
  k_1/1(Out1) -> Product1/1
  k_0/1(Out1) -> Add/1
  [insan] -> k_1/1(In1), k_0/1(In1), Divide7/1

== system HMC/Reference CVSs/eRV/eRV2 ==
  note: y = 0,005x 2 + 0,25x + 17
  Add18 : Sum
  Add19 : Sum
  Constant20 : Constant  Value=17
  Gain1 : Gain  Gain=1/100
  Gain2 : Gain  Gain=0.005
  Gain3 : Gain  Gain=0.25
  PID : Subsystem  Commented=on
  Product15 : Product
  Scope : Scope
      settings: ActiveDisplayYMinimum=1.07059  ActiveDisplayYMaximum=1.42514
  Stair Generator : powerlib_meascontrol/Pulse & Signal Generators/Stair Generator  Commented=on  t=[0,50,100,150]  e=[3.25,3.5,3.75,4]  Ts=stepsize
      settings: SourceProductName=Simscape Electrical
  Stair Generator1 : powerlib_meascontrol/Pulse & Signal Generators/Stair Generator  Commented=on  t=[100,200,300,400]  e=[3.25,3.5,3.75,4]  Ts=stepsize
      settings: SourceProductName=Simscape Electrical
  Output : Outport
  wires:
  Gain1/1 -> Output/1, Scope/1
  Constant20/1 -> Add19/2
  Product15/1 -> Gain2/1
  Add18/1 -> Add19/1
  [HR] -> Gain3/1, Product15/2, Product15/1
  Gain3/1 -> Add18/2
  Gain2/1 -> Add18/1
  Add19/1 -> Gain1/1
  Stair Generator1/1 -> PID/1(s)

== system HMC/Reference CVSs/eRV/eRVhf ==
  note: y = 0,0056x 2 - 0,6667x + 60
  Add18 : Sum
  Add19 : Sum
  Constant20 : Constant  Value=60
  Gain1 : Gain  Gain=1/100
  Gain2 : Gain  Gain=0.0056
  Gain3 : Gain  Gain=-0.6667
  PID : Subsystem  Commented=on
  Product15 : Product
  Scope : Scope
      settings: ActiveDisplayYMinimum=1.07059  ActiveDisplayYMaximum=1.42514
  Stair Generator : powerlib_meascontrol/Pulse & Signal Generators/Stair Generator  Commented=on  t=[0,50,100,150]  e=[3.25,3.5,3.75,4]  Ts=stepsize
      settings: SourceProductName=Simscape Electrical
  Stair Generator1 : powerlib_meascontrol/Pulse & Signal Generators/Stair Generator  Commented=on  t=[100,200,300,400]  e=[3.25,3.5,3.75,4]  Ts=stepsize
      settings: SourceProductName=Simscape Electrical
  Output : Outport
  wires:
  Gain1/1 -> Output/1, Scope/1
  Constant20/1 -> Add19/2
  Product15/1 -> Gain2/1
  Add18/1 -> Add19/1
  [HR] -> Gain3/1, Product15/2, Product15/1
  Gain3/1 -> Add18/2
  Gain2/1 -> Add18/1
  Add19/1 -> Gain1/1
  Stair Generator1/1 -> PID/1(s)

== system HMC/IBS_LVAD/Subsystem1/QA REF/Gain Regulator ==
  Add : Sum  Inputs=+-
  Add1 : Sum  Inputs=+++
  Constant1 : Constant  Value=83.5
  Constant2 : Constant  Value=-100
  Display : Display
  Gain1 : Gain  Gain=1.2
  Gain2 : Gain  Gain=-2.6667
  Gain3 : Gain  Gain=0.0444
  Gain4 : Gain  Gain=0.1
  Product : Product
  Switch1 : Switch  Threshold=1  SaturateOnIntegerOverflow=off  InputSameDT=off
  Out1 : Outport  VectorParamsAs1DForOutWhenUnconnected=off
  wires:
  Gain1/1 -> Add/1
  [HR] -> Gain1/1
  Constant1/1 -> Add/2
  Add/1 -> Switch1/1
  [Exercise_On_Off] -> Switch1/2
  [insan] -> Product/2, Gain2/1, Product/1
  Product/1 -> Gain3/1
  Constant2/1 -> Add1/3
  Gain2/1 -> Add1/2
  Gain3/1 -> Add1/1
  Add1/1 -> Gain4/1
  Gain4/1 -> Switch1/3
  Switch1/1 -> Out1/1, Display/1

== system HMC/IBS_LVAD/Subsystem1/QA REF/Subsystem18 ==
  In1 : Inport
  Add1 : Sum
  Product3 : Product
  Product4 : Product
  Sin : Trigonometry
  a1 : Constant  Value=6.408
  "b1 " : Constant  Value=3.677
  c1 : Constant  Value=1.495
  Out1 : Outport  VectorParamsAs1DForOutWhenUnconnected=off
  wires:
  c1/1 -> Add1/2
  Product3/1 -> Add1/1
  Add1/1 -> Sin/1
  a1/1 -> Product4/2
  "b1 "/1 -> Product3/2
  Product4/1 -> Out1/1
  Sin/1 -> Product4/1
  In1/1 -> Product3/1

== system HMC/IBS_LVAD/Subsystem1/QA REF/Subsystem19 ==
  In1 : Inport
  Add1 : Sum
  Product3 : Product
  Product4 : Product
  Sin : Trigonometry
  a1 : Constant  Value=79.1
  "b1 " : Constant  Value=0.004367
  c1 : Constant  Value=1.947
  Out1 : Outport  VectorParamsAs1DForOutWhenUnconnected=off
  wires:
  c1/1 -> Add1/2
  Product3/1 -> Add1/1
  Add1/1 -> Sin/1
  a1/1 -> Product4/2
  "b1 "/1 -> Product3/2
  Product4/1 -> Out1/1
  Sin/1 -> Product4/1
  In1/1 -> Product3/1

== system HMC/IBS_LVAD/Subsystem1/QA REF/Subsystem20 ==
  In1 : Inport
  Add1 : Sum
  Product3 : Product
  Product4 : Product
  Sin : Trigonometry
  a1 : Constant  Value=12.51
  "b1 " : Constant  Value=0.9098
  c1 : Constant  Value=-0.7412
  Out1 : Outport  VectorParamsAs1DForOutWhenUnconnected=off
  wires:
  In1/1 -> Product3/1
  Sin/1 -> Product4/1
  Product4/1 -> Out1/1
  "b1 "/1 -> Product3/2
  a1/1 -> Product4/2
  Add1/1 -> Sin/1
  Product3/1 -> Add1/1
  c1/1 -> Add1/2

== system HMC/IBS_LVAD/Subsystem1/QA REF/Subsystem21 ==
  In1 : Inport
  Add1 : Sum
  Product3 : Product
  Product4 : Product
  Sin : Trigonometry
  a1 : Constant  Value=9.82
  "b1 " : Constant  Value=1.804
  c1 : Constant  Value=0.09731
  Out1 : Outport  VectorParamsAs1DForOutWhenUnconnected=off
  wires:
  c1/1 -> Add1/2
  Product3/1 -> Add1/1
  Add1/1 -> Sin/1
  a1/1 -> Product4/2
  "b1 "/1 -> Product3/2
  Product4/1 -> Out1/1
  Sin/1 -> Product4/1
  In1/1 -> Product3/1

== system HMC/IBS_LVAD/Subsystem1/QA REF/Subsystem22 ==
  In1 : Inport
  Add1 : Sum
  Product3 : Product
  Product4 : Product
  Sin : Trigonometry
  a1 : Constant  Value=8.175
  "b1 " : Constant  Value=2.741
  c1 : Constant  Value=0.7476
  Out1 : Outport  VectorParamsAs1DForOutWhenUnconnected=off
  wires:
  In1/1 -> Product3/1
  Sin/1 -> Product4/1
  Product4/1 -> Out1/1
  "b1 "/1 -> Product3/2
  a1/1 -> Product4/2
  Add1/1 -> Sin/1
  Product3/1 -> Add1/1
  c1/1 -> Add1/2

== system HMC/IBS_LVAD/Subsystem1/Subsystem/HeartRate1 ==
  Display : Display
  Display1 : Display
  Display2 : Display
  Switch2 : Switch  Criteria=u2 > Threshold  SaturateOnIntegerOverflow=off  InputSameDT=off
  Out1 : Outport
  tag scope: insann=global
  wires:
  [HR_REF] -> Out1/1, Switch2/1, Display/1
  [Exercise_REF] -> Switch2/2
  [Non_exercise_HR_REF] -> Display1/1, Switch2/3
  Switch2/1 -> [insann], Display2/1

== system HMC/IBS_LVAD/Subsystem1/Subsystem/Pm1 ==
  note: y = -0,3333x2 + 116,67x - 5800R² = 1
  note: y = -0,0333x 2 + 11,667x - 580
  Add18 : Sum
  Add19 : Sum
  Constant20 : Constant  Value=-580
  Gain1 : Gain  Gain=1/100
  Gain2 : Gain  Gain=-0.0333
  Gain3 : Gain  Gain=11.667
  PID : Subsystem  Commented=on
  Product15 : Product
  Scope : Scope
      settings: ActiveDisplayYMinimum=3.007  ActiveDisplayYMaximum=5.007
  tag scope: PMM=global
  wires:
  Add19/1 -> Gain1/1
  Gain2/1 -> Add18/1
  Gain3/1 -> Add18/2
  [HR] -> Product15/1, Product15/2, Gain3/1
  Add18/1 -> Add19/1
  Product15/1 -> Gain2/1
  Constant20/1 -> Add19/2
  Gain1/1 -> [PMM], Scope/1

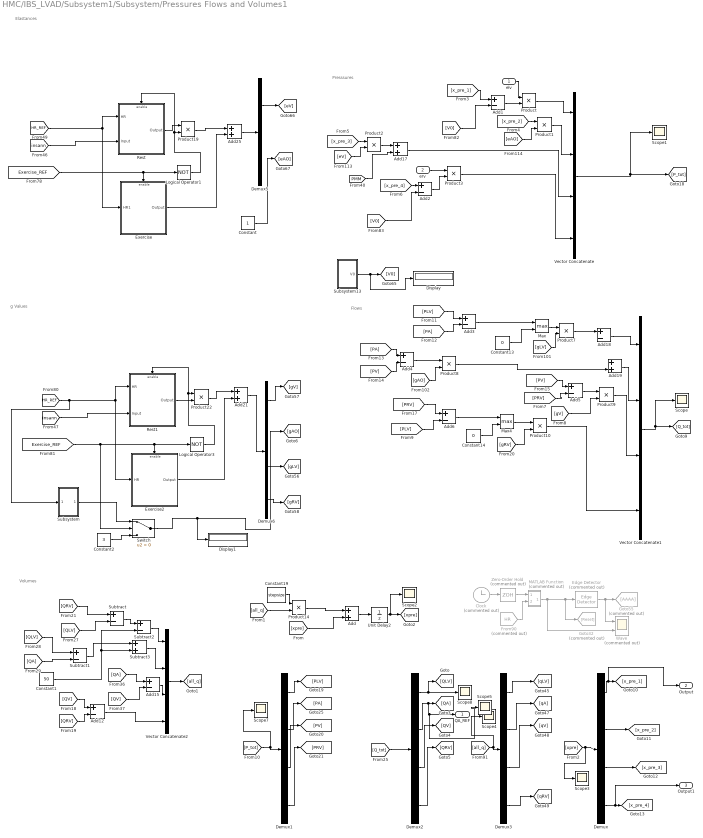
== system HMC/IBS_LVAD/Subsystem1/Subsystem/Pressures Flows and Volumes1 ==
  note: Volumes
  note: Flows
  note: Presssures
  note: g Values
  note: Elastances
  elv : Inport
  erv : Inport  Port=2
  Add{,17,19,21,25} (5 alike) : Sum
  Add{1..6,12,15,18} (9 alike) : Sum  Inputs=+-
  Clock : Clock  Commented=on
      settings: Decimation=10000000
  Constant : Constant
  Constant1 : Constant  Value=50
  Constant13 : Constant  Value=0
  Constant14 : Constant  Value=0
  Constant19 : Constant  Value=stepsize
  Constant2 : Constant  Value=3
  Demux{,1..3,6} (5 alike) : Demux
  Demux5 : Demux  Outputs=2
  Display : Display
  Display1 : Display
  Edge Detector : powerlib_meascontrol/Logic/Edge Detector  Commented=on  model=Falling  ic=0  Ts=0
      settings: SourceProductName=Simscape Electrical
  Exercise : Subsystem  TreatAsAtomicUnit=on
  Exercise2 : Subsystem  TreatAsAtomicUnit=on
  From90 : From  Commented=on  GotoTag=HR  TagVisibility=global
  Goto32 : Goto  Commented=on  GotoTag=Reset
  Goto55 : Goto  Commented=on  GotoTag=AAAA
  Logical Operator1 : Logic  Operator=NOT  AllPortsSameDT=off  OutDataTypeStr=boolean
  Logical Operator3 : Logic  Operator=NOT  AllPortsSameDT=off  OutDataTypeStr=boolean
  MATLAB Function : MATLAB Function  Commented=on  TreatAsAtomicUnit=on
  Max : MinMax  Function=max  Inputs=2
  Max4 : MinMax  Function=max  Inputs=2
  Product{,1..3,7..10,14,19,22} (11 alike) : Product
  Rest : Subsystem  TreatAsAtomicUnit=on
  Rest1 : Subsystem  TreatAsAtomicUnit=on
  Scope{,1..5,7..8} (8 alike) : Scope
      Scope settings: ActiveDisplayYMinimum=-77.48033  ActiveDisplayYMaximum=390.18057  DataLoggingVariableName=ScopeData3
      Scope1 settings: ActiveDisplayYMinimum=-17.90547  ActiveDisplayYMaximum=127.32097  DataLoggingVariableName=ScopeData4
      Scope2 settings: ActiveDisplayYMinimum=-34.04375  ActiveDisplayYMaximum=306.39376  DataLoggingVariableName=ScopeData3
      Scope3 settings: ActiveDisplayYMinimum=-369.57927  ActiveDisplayYMaximum=469.20086  DataLoggingVariableName=ScopeData3
      Scope4 settings: ActiveDisplayYMinimum=-3614.79854  ActiveDisplayYMaximum=3696.63533
      Scope5 settings: ActiveDisplayYMinimum=-56.09763  ActiveDisplayYMaximum=71.61871
      Scope7 settings: ActiveDisplayYMinimum=-6.49879  ActiveDisplayYMaximum=43.7952  DataLoggingVariableName=ScopeData3
      Scope8 settings: ActiveDisplayYMinimum=-106.50454  ActiveDisplayYMaximum=958.54088  DataLoggingVariableName=ScopeData10
  Subsystem : Subsystem
  Subsystem13 : Subsystem
  Subtract : Sum  Inputs=+-
  Subtract1 : Sum  Inputs=+-
  Subtract2 : Sum  Inputs=+-
  Subtract3 : Sum
  Switch : Switch  Criteria=u2 > Threshold  SaturateOnIntegerOverflow=off  InputSameDT=off
  Unit Delay2 : UnitDelay  InitialCondition=X_00  SampleTime=-1
  Vector Concatenate : Concatenate  NumInputs=4
  Vector Concatenate1 : Concatenate  NumInputs=4
  Vector Concatenate2 : Concatenate  NumInputs=4
  Wave : Scope  Commented=on  NumInputPorts=2
      settings: ActiveDisplayYMinimum=-0.125  ActiveDisplayYMaximum=1.125  DataLoggingVariableName=ScopeData2
  Zero-Order Hold : ZeroOrderHold  Commented=on  SampleTime=-1
  QA_REF : Outport  VectorParamsAs1DForOutWhenUnconnected=off
  Output : Outport  Port=2
  Output1 : Outport  Port=3
  wires:
  Product14/1 -> Add/1
  [xpre] -> Add/2
  elv/1 -> Product/1
  [xpre] -> Scope3/1, Demux/1
  Demux/3 -> [x_pre_3]
  [x_pre_1] -> Add1/1
  Add1/1 -> Product/2
  Product/1 -> Vector Concatenate/1
  [x_pre_2] -> Product1/1
  Product1/1 -> Vector Concatenate/2
  Add2/1 -> Product3/2
  Product3/1 -> Vector Concatenate/4
  erv/1 -> Product3/1
  [P_tot] -> Scope7/1, Demux1/1
  Demux1/1 -> [PLV]
  Demux1/4 -> [PRV]
  Demux1/3 -> [PV]
  [PLV] -> Add3/1
  [PA] -> Add3/2
  Max/1 -> Product7/1
  [PA] -> Add4/1
  [PV] -> Add4/2
  Add4/1 -> Product8/1
  [PV] -> Add5/1
  [PRV] -> Add5/2
  Add5/1 -> Product9/1
  Constant14/1 -> Max4/2
  [PRV] -> Add6/1
  [PLV] -> Add6/2
  Max4/1 -> Product10/1
  Product10/1 -> Vector Concatenate1/4
  Demux2/1 -> Scope8/1, [QLV]
  Demux2/3 -> [QV]
  Demux2/2 -> [QA], Scope5/1, QA_REF/1
  [QRV] -> Subtract/1
  [QLV] -> Subtract1/1
  [QA] -> Subtract1/2
  [QV] -> Add12/1
  [QRV] -> Add12/2
  [QA] -> Add15/1
  [QV] -> Add15/2
  Vector Concatenate/1 -> [P_tot], Scope1/1
  Vector Concatenate1/1 -> [Q_tot], Scope/1
  Vector Concatenate2/1 -> [all_q]
  [all_q] -> Product14/2
  Product2/1 -> Add17/1
  Add17/1 -> Vector Concatenate/3
  Add6/1 -> Max4/1
  Add3/1 -> Max/1
  Constant13/1 -> Max/2
  [x_pre_3] -> Product2/1
  [x_pre_4] -> Add2/1
  Add15/1 -> Vector Concatenate2/3
  Add12/1 -> Vector Concatenate2/4
  Constant19/1 -> Product14/1
  Add/1 -> Unit Delay2/1
  Unit Delay2/1 -> Scope2/1, [xpre]
  [Q_tot] -> Demux2/1
  Product9/1 -> Vector Concatenate1/3
  [QLV] -> Subtract/2
  Clock/1 -> Zero-Order Hold/1
  Zero-Order Hold/1 -> MATLAB Function/1(u)
  Demux3/1 -> [qLV]
  Demux3/2 -> [qA]
  Demux3/3 -> [qV]
  Demux3/4 -> [qRV]
  Edge Detector/1 -> Wave/1, Goto55/1
  [gLV] -> Product7/2
  [gAO] -> Product8/2
  [gV] -> Product9/2
  [gRV] -> Product10/2
  [V0] -> Add1/2
  [V0] -> Add2/2
  [eV] -> Product2/2
  [eAO] -> Product1/2
  Product7/1 -> Add18/1
  Add18/1 -> Vector Concatenate1/1
  Product8/1 -> Add19/2
  Add19/1 -> Vector Concatenate1/2
  Demux1/2 -> [PA]
  MATLAB Function/1(y) -> Wave/2, Edge Detector/1, Goto32/1
  From90/1 -> MATLAB Function/2(HR)
  Demux/2 -> [x_pre_2]
  [all_q] -> Scope4/1, Demux3/1
  Demux2/4 -> [QRV]
  [PMM] -> Add17/2
  Demux/4 -> [x_pre_4], Output1/1
  Demux/1 -> [x_pre_1], Output/1
  [insann] -> Rest1/2(Input)
  Rest1/1(Output) -> Product22/2
  Demux5/1 -> [eV]
  Exercise2/1(Output) -> Add21/2
  Logical Operator3/1 -> Product22/1, Rest1/Enable
  Exercise/1(Output) -> Add25/2
  Product22/1 -> Add21/1
  [insann] -> Rest/2(Input)
  Demux6/1 -> [gV]
  Add21/1 -> Demux6/1
  Demux6/3 -> [gLV]
  [HR_REF] -> Exercise/1(HR1), Rest/1(HR)
  Add25/1 -> Demux5/1
  [Exercise_REF] -> Logical Operator3/1, Exercise2/Enable, Switch/2
  Rest/1(Output) -> Product19/1
  Demux6/4 -> [gRV]
  Logical Operator1/1 -> Product19/2, Rest/Enable
  Product19/1 -> Add25/1
  [Exercise_REF] -> Logical Operator1/1, Exercise/Enable
  [HR_REF] -> Subsystem/1(In1), Exercise2/1(HR), Rest1/1(HR)
  Subsystem13/1(V0) -> Display/1, [V0]
  Constant/1 -> [eAO]
  Switch/1 -> [gAO], Display1/1
  Constant2/1 -> Switch/3
  Subsystem/1(Out1) -> Switch/1
  Constant1/1 -> Subtract3/2, Subtract2/2
  Subtract/1 -> Subtract2/1
  Subtract2/1 -> Vector Concatenate2/1
  Subtract1/1 -> Subtract3/1
  Subtract3/1 -> Vector Concatenate2/2

== system HMC/IBS_LVAD/Subsystem1/Subsystem/eLV1 ==
  VLV : Inport
  HR : Inport  Port=2
  Clock1 : Clock
  Constant : Constant  Value=3
  LV_e_min : Subsystem
  Scope : Scope
      settings: ActiveDisplayYMinimum=-0.72024  ActiveDisplayYMaximum=3.41705
  Subsystem1 : Subsystem
  Switch1 : Switch  Criteria=u2 > Threshold  Threshold=0.9  SaturateOnIntegerOverflow=off  InputSameDT=off
  eLV1 : Subsystem
  elv : Outport
  tag scope: eLVV=global
  wires:
  Clock1/1 -> Subsystem1/4(t)
  Subsystem1/1(elv) -> Scope/1, elv/1
  VLV/1 -> LV_e_min/1(VLV)
  HR/1 -> Subsystem1/3(HR)
  LV_e_min/1(eLV_min_O) -> Subsystem1/2(eLV_min)
  Constant/1 -> Switch1/3
  [Exercise_REF] -> Switch1/2
  eLV1/1(Output) -> Switch1/1
  Switch1/1 -> Subsystem1/1(eLV_max), [eLVV]

== system HMC/IBS_LVAD/Subsystem1/Subsystem/eRV1 ==
  HR : Inport
  VRV : Inport  Port=2
  Clock2 : Clock
  Display : Display
  RV_e_min : Subsystem
  Subsystem2 : Subsystem
  eRV2 : Subsystem
  eRV1 : Outport
  tag scope: eRVV=global
  wires:
  Clock2/1 -> Subsystem2/3(t)
  HR/1 -> Subsystem2/4(HR)
  VRV/1 -> RV_e_min/1(VRV)
  Subsystem2/1(eRV) -> eRV1/1
  RV_e_min/1(eRV_min_O) -> Subsystem2/2(eRV_min)
  eRV2/1(Output) -> Subsystem2/1(eRV_max), Display/1, [eRVV]

== system HMC/RTI Data/RTI Data Store/RTI Data Store/RTI Data Store ==
  RTI Data Store : Subsystem  mask(RTI_DATA_STORE){}
      mask help:
      | RTI Data Store Block. This block is used by RTI to store internal model dependent data. Deleting this block will result in data loss.
      |
      | NEVER DELETE, COPY, OR MODIFY THIS BLOCK!
      mask Help:
      | RTI Data Store Block. This block is used by RTI to store internal model dependent data. Deleting this block will result in data loss.
      | 
      | NEVER DELETE, COPY, OR MODIFY THIS BLOCK!
      mask Display: text(0.5, 0.5, ' ', 'HorizontalAlignment', 'center');

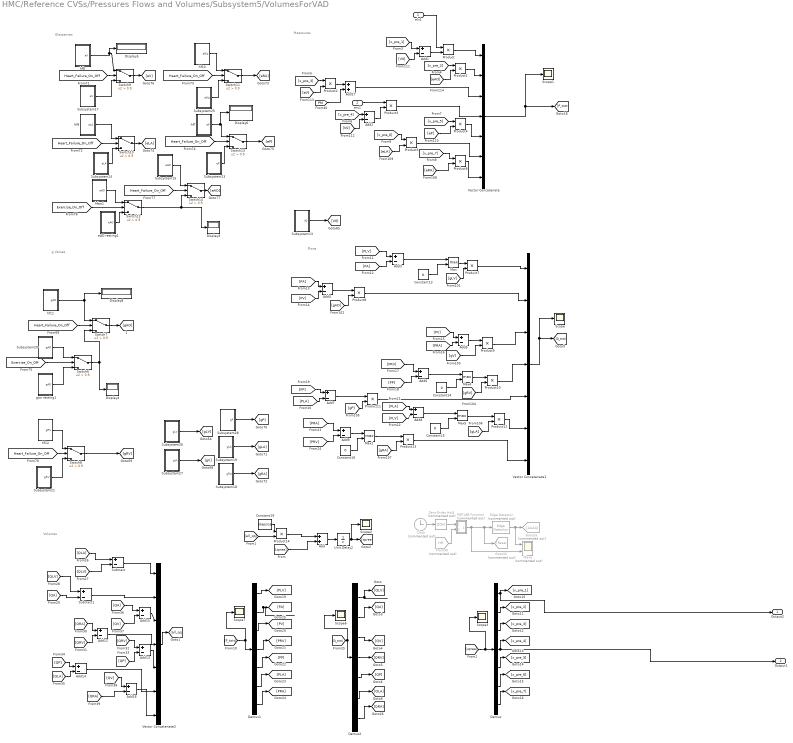
== system HMC/Reference CVSs/Pressures Flows and Volumes/Subsystem5/VolumesForVAD ==
  note: Volumes
  note: Flows
  note: g Values
  note: Presssures
  note: Elastances
  elv1 : Inport
  erv1 : Inport  Port=2
  Add : Sum
  Add{1..9,12..16} (14 alike) : Sum  Inputs=+-
  Add17 : Sum
  Clock : Clock  Commented=on
      settings: Decimation=10000000
  Constant{13..16} (4 alike) : Constant  Value=0
  Constant19 : Constant  Value=stepsize
  Demux : Demux  Outputs=7
  Demux1 : Demux  Outputs=7
  Demux2 : Demux  Outputs=7
  Display{3..6,8} (5 alike) : Display
  Edge Detector : powerlib_meascontrol/Logic/Edge Detector  Commented=on  model=Falling  ic=0  Ts=0
      settings: SourceProductName=Simscape Electrical
  From90 : From  Commented=on  GotoTag=HR  TagVisibility=global
  Goto32 : Goto  Commented=on  GotoTag=Reset
  Goto55 : Goto  Commented=on  GotoTag=AAAA
  MATLAB Function : MATLAB Function  Commented=on  TreatAsAtomicUnit=on
  Max{,1,4..5} (4 alike) : MinMax  Function=max  Inputs=2
  Product{,1..14} (15 alike) : Product
  Scope{,1..3,6..7} (6 alike) : Scope
      Scope settings: ActiveDisplayYMinimum=-554.9505  ActiveDisplayYMaximum=4972.61734
      Scope1 settings: ActiveDisplayYMinimum=60.37603  ActiveDisplayYMaximum=117.27305  DataLoggingVariableName=ScopeData2
      Scope2 settings: ActiveDisplayYMinimum=-34.04375  ActiveDisplayYMaximum=306.39376  DataLoggingVariableName=ScopeData4
      Scope3 settings: ActiveDisplayYMinimum=-652.22865  ActiveDisplayYMaximum=5628.02541  DataLoggingVariableName=ScopeData5
      Scope6 settings: ActiveDisplayYMinimum=-1063.20433  ActiveDisplayYMaximum=9460.42216  DataLoggingVariableName=ScopeData7
      Scope7 settings: ActiveDisplayYMinimum=-11.3052  ActiveDisplayYMaximum=174.2221  DataLoggingVariableName=ScopeData8
  Subsystem13 : Subsystem
  Subsystem15 : Subsystem
  Subsystem17 : Subsystem
  Subsystem18 : Subsystem
  Subsystem19 : Subsystem
  Subsystem20 : Subsystem
  Subsystem21 : Subsystem
  Subsystem23 : Subsystem
  Subsystem24 : Subsystem
  Subsystem25 : Subsystem
  Subsystem26 : Subsystem
  Subsystem27 : Subsystem
  Subsystem28 : Subsystem
  Subtract : Sum  Inputs=+-
  Subtract1 : Sum  Inputs=+-
  Switch{6..14} (9 alike) : Switch  Criteria=u2 > Threshold  Threshold=0.9  SaturateOnIntegerOverflow=off  InputSameDT=off
  Unit Delay2 : UnitDelay  InitialCondition=X_0  SampleTime=-1
  Vector Concatenate : Concatenate  NumInputs=7
  Vector Concatenate1 : Concatenate  NumInputs=7
  Vector Concatenate2 : Concatenate  NumInputs=7
  Wave : Scope  Commented=on  NumInputPorts=2
      settings: ActiveDisplayYMinimum=-0.125  ActiveDisplayYMaximum=1.125  DataLoggingVariableName=ScopeData10
  Zero-Order Hold : ZeroOrderHold  Commented=on  SampleTime=-1
  eAO resting1 : Subsystem
  gao resting1 : Subsystem
  hf10 : Subsystem
  hf11 : Subsystem
  hf12 : Subsystem
  hf7 : Subsystem
  hf8 : Subsystem
  hf9 : Subsystem
  hfao1 : Subsystem
  Output2 : Outport
  Output1 : Outport  Port=2
  wires:
  Demux1/3 -> [PV]
  hf7/1(eP) -> Display6/1, Switch13/1
  [QRV] -> Add12/2
  [gLV] -> Product7/2
  Constant16/1 -> Max1/2
  hf9/1(eLA) -> Switch10/1
  [Exercise_On_Off] -> Switch6/2
  [Q_tott] -> Demux2/1, Scope6/1
  Add2/1 -> Product3/2
  Constant14/1 -> Max4/2
  [eAO] -> Product1/2
  [PP] -> Add7/1
  Subsystem25/1(eRA) -> Switch11/3
  [Heart_Failure_On_Off] -> Switch11/2
  [V0] -> Add1/2
  Product6/1 -> Vector Concatenate/7
  eAO resting1/1(eAO) -> Switch12/3
  Demux2/3 -> [QV]
  Subtract/1 -> Vector Concatenate2/1
  [Exercise_On_Off] -> Switch12/2
  [QLA] -> Add14/2
  hf10/1(eRA) -> Switch11/1
  [PM] -> Add17/2
  Product1/1 -> Vector Concatenate/2
  Subsystem28/1(gP) -> [gP]
  [xpree] -> Scope3/1, Demux/1
  Switch7/1 -> [gAO]
  Subsystem18/1(gRA) -> [gRA]
  Switch8/1 -> [gRV]
  Switch14/1 -> [eAO]
  [all_qq] -> Product14/2
  Add7/1 -> Product11/1
  Subsystem20/1(gAO) -> Switch6/1
  [eLA] -> Product5/2
  Subsystem17/1(eV) -> Switch9/3
  Subsystem23/1(eP) -> Switch13/3
  hf11/1(gAO) -> Display8/1, Switch7/1
  [Heart_Failure_On_Off] -> Switch8/2
  [PLA] -> Add7/2
  ? -> ?
  [PA] -> Add3/2
  Subsystem24/1(eLA) -> Switch10/3
  Constant19/1 -> Product14/1
  [QP] -> Add14/1
  Demux/5 -> [x_pre_5]
  Switch6/1 -> Switch7/3, Display4/1
  gao resting1/1(gAO) -> Switch6/3
  Product7/1 -> Vector Concatenate1/1
  Switch12/1 -> Display3/1, Switch14/3
  Switch11/1 -> [eRA]
  [Heart_Failure_On_Off] -> Switch13/2
  Demux/4 -> [x_pre_4], Output1/1
  Add3/1 -> Max/1
  [x_pre_2] -> Product1/1
  [Heart_Failure_On_Off] -> Switch9/2
  Switch10/1 -> [eLA]
  Clock/1 -> Zero-Order Hold/1
  Switch13/1 -> [eP]
  [gV] -> Product9/2
  [PV] -> Add4/2
  [QP] -> Add13/2
  [PRA] -> Add5/2
  Subtract1/1 -> Vector Concatenate2/2
  [PRV] -> Add9/2
  Demux1/5 -> [PP]
  Add14/1 -> Vector Concatenate2/6
  Add4/1 -> Product8/1
  Subsystem26/1(gLV) -> [gLV]
  Demux/2 -> [x_pre_2]
  Subsystem27/1(gVt) -> [gV]
  Subsystem15/1(eAO) -> Switch14/1
  Subsystem13/1(V0) -> [V0]
  hf8/1(eV) -> Display5/1, Switch9/1
  [PRA] -> Add9/1
  Demux/1 -> [x_pre_1], Output2/1
  Demux/6 -> [x_pre_6]
  Edge Detector/1 -> Wave/1, Goto55/1
  Max4/1 -> Product10/1
  Add16/1 -> Vector Concatenate2/7
  hfao1/1(eAO) -> Switch12/1
  Demux2/4 -> [QRV]
  Demux2/5 -> [QP]
  Add15/1 -> Vector Concatenate2/3
  Zero-Order Hold/1 -> MATLAB Function/1(u)
  Vector Concatenate2/1 -> [all_qq]
  Demux2/7 -> [QRA]
  Add8/1 -> Max5/1
  Demux/7 -> [x_pre_7]
  Product8/1 -> Vector Concatenate1/2
  [gRV] -> Product10/2
  Switch9/1 -> [eV]
  [x_pre_5] -> Product4/1
  From90/1 -> MATLAB Function/2(HR)
  Product5/1 -> Vector Concatenate/6
  MATLAB Function/1(y) -> Wave/2, Edge Detector/1, Goto32/1
  Max/1 -> Product7/1
  [gP] -> Product11/2
  [xpree] -> Add/2
  [eRA] -> Product6/2
  [eV] -> Product2/2
  [gRA] -> Product13/2
  [gLA] -> Product12/2
  Product12/1 -> Vector Concatenate1/6
  Vector Concatenate1/1 -> [Q_tott], Scope/1
  [gAO] -> Product8/2
  [V0] -> Add2/2
  [eP] -> Product4/2
  Product3/1 -> Vector Concatenate/4
  [QLV] -> Subtract/2
  [x_pre_3] -> Product2/1
  hf12/1(gRV) -> Switch8/1
  Add12/1 -> Vector Concatenate2/4
  Unit Delay2/1 -> Scope2/1, [xpree]
  Vector Concatenate/1 -> [P_tott], Scope1/1
  Product2/1 -> Add17/1
  Product9/1 -> Vector Concatenate1/3
  [Heart_Failure_On_Off] -> Switch14/2
  Add17/1 -> Vector Concatenate/3
  Add13/1 -> Vector Concatenate2/5
  [Heart_Failure_On_Off] -> Switch10/2
  [QLV] -> Subtract1/1
  Subsystem19/1(gLA) -> [gLA]
  Max1/1 -> Product13/1
  [QLA] -> Subtract/1
  [QRA] -> Add16/2
  [x_pre_1] -> Add1/1
  Demux2/1 -> [QLV]
  erv1/1 -> Product3/1
  [x_pre_6] -> Product5/1
  [QA] -> Subtract1/2
  [x_pre_4] -> Add2/1
  [PV] -> Add5/1
  Add6/1 -> Max4/1
  [PLA] -> Add8/1
  Product11/1 -> Vector Concatenate1/5
  Subsystem21/1(gRV) -> Switch8/3
  Add5/1 -> Product9/1
  Product10/1 -> Vector Concatenate1/4
  [QV] -> Add15/2
  [Heart_Failure_On_Off] -> Switch7/2
  [QRA] -> Add12/1
  Demux1/1 -> [PLV]
  [PA] -> Add4/1
  [PRV] -> Add6/1
  Demux1/7 -> [PRA]
  Max5/1 -> Product12/1
  [PLV] -> Add3/1
  Constant15/1 -> Max5/2
  [PLV] -> Add8/2
  [QV] -> Add16/1
  Constant13/1 -> Max/2
  Product/1 -> Vector Concatenate/1
  Demux2/6 -> [QLA]
  elv1/1 -> Product/1
  Add9/1 -> Max1/1
  Product14/1 -> Add/1
  Demux1/4 -> [PRV]
  Demux2/2 -> [QA]
  [PP] -> Add6/2
  Demux1/6 -> [PLA]
  Product13/1 -> Vector Concatenate1/7
  [x_pre_7] -> Product6/1
  Demux/3 -> [x_pre_3]
  [QRV] -> Add13/1
  [P_tott] -> Scope7/1, Demux1/1
  Add1/1 -> Product/2
  [QA] -> Add15/1
  Product4/1 -> Vector Concatenate/5
  Demux1/2 -> [PA]
  Add/1 -> Unit Delay2/1
